simulink model "ToyModel_Bus"  (R2018b)
settings: Solver=ode1  StartTime=0.0  StopTime=10.0  FixedStep=0.001  RelTol=1e-3
libraries: simulink x1
settings Model: Creator=ogihara  LastModifiedBy=ogihara

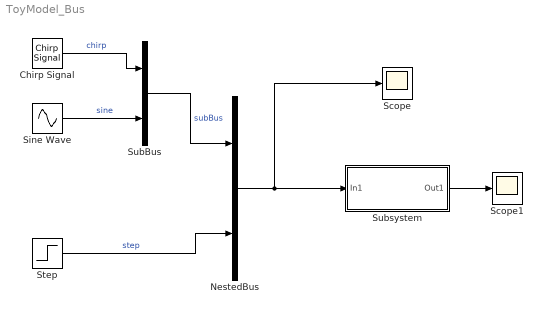
== system ToyModel_Bus ==
  Chirp Signal : simulink/Sources/Chirp Signal  f1=0.1  T=10  f2=1
  NestedBus : BusCreator  Inputs=2
  Scope : Scope
  Scope1 : Scope
  Sine Wave : Sin  Amplitude=0.5  SampleTime=0
  Step : Step  Time=3  SampleTime=0
  "SubBus " : BusCreator  Inputs=2
  Subsystem : Subsystem
  wires:
  Chirp Signal/1 -> "SubBus "/1  "chirp"
  Sine Wave/1 -> "SubBus "/2  "sine"
  "SubBus "/1 -> NestedBus/1  "subBus"
  Step/1 -> NestedBus/2  "step"
  NestedBus/1 -> Subsystem/1(In1), Scope/1
  Subsystem/1(Out1) -> Scope1/1

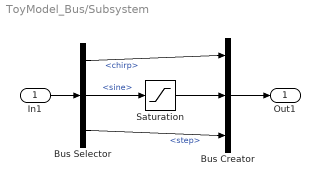
== system ToyModel_Bus/Subsystem ==
  In1 : Inport
  Bus Creator : BusCreator  Inputs=3
  Bus Selector : BusSelector  OutputSignals=subBus.chirp,subBus.sine,step
  Saturation : Saturate  UpperLimit=0.3
  Out1 : Outport
  wires:
  In1/1 -> Bus Selector/1
  Bus Selector/2 -> Saturation/1  "<sine>"
  Bus Selector/3 -> Bus Creator/3  "<step>"
  Bus Creator/1 -> Out1/1
  Bus Selector/1 -> Bus Creator/1  "<chirp>"
  Saturation/1 -> Bus Creator/2
